simulink model "crop_simulation"  (R2021a)
settings: Solver=ode23tb  StartTime=0.0  StopTime=4  RelTol=1e-2
values from neighbouring files (symbols this model uses):
  parameters = LoadParameters()    [OnlyPlots.m]    (also in run_crop_simulation.m; run_several_crop_simulation.m)
undefined symbols (not defined in the file or in its folder): climate_GH3, MM_vec, nearst_p, p, PowerArtificial, Tr, Tref, Ts, x0_SOFC
libraries: HORTISIM x14, pid_lib x4
(part 2 of 3)

== system crop_simulation/Control Systems/Heater/SOFC/Subsystem2/Subsystem2 ==
  EPD : Inport
  Target : Inport  Port=2
  MATLAB Function : MATLAB Function  TreatAsAtomicUnit=on
  Memory : Memory
  Memory1 : Memory
  Rate Limiter : RateLimiter  RisingSlewLimit=5000  FallingSlewLimit=-5000
  Rate Transition : RateTransition  OutPortSampleTime=1/(60*24)
  Rate Transition1 : RateTransition  OutPortSampleTime=0
  Scope : Scope  NumInputPorts=3
  Vector Concatenate : Concatenate
  I [A] : Outport
  wires:
  MATLAB Function/1(y) -> Scope/2, Rate Transition1/1, Memory1/1
  EPD/1 -> Vector Concatenate/2, Memory/1
  Memory/1 -> Rate Transition/1
  Target/1 -> Vector Concatenate/1, MATLAB Function/1(Target)
  Rate Transition/1 -> MATLAB Function/2(FPD)
  Memory1/1 -> MATLAB Function/3(upre)
  Vector Concatenate/1 -> Scope/1
  Rate Limiter/1 -> Scope/3, I [A]/1
  Rate Transition1/1 -> Rate Limiter/1

== system crop_simulation/Control Systems/Heater/SOFC/Water Tank /Control Law ==
  Ti : Inport
  Tw : Inport  Port=2
  Constant : Constant  Value=273.15
  Control Flow Rate [%] : Subsystem
  Gain1 : Gain  Gain=90
  Minus : Sum  Inputs=+-
  Product : Product
  Scope2 : Scope
  Sum : Sum  Inputs=|++
  Heat[W] : Outport
  wires:
  Product/1 -> Heat[W]/1
  Tw/1 -> Minus/2
  Control Flow Rate [%]/1(Out1) -> Scope2/1, Product/2
  Gain1/1 -> Product/1
  Minus/1 -> Gain1/1
  Ti/1 -> Control Flow Rate [%]/1(Ti), Sum/1
  Sum/1 -> Minus/1
  Constant/1 -> Sum/2

== system crop_simulation/Control Systems/Heater/SOFC/Water Tank /recooling ==
  Tw : Inport
  Constant : Constant  Value=273.15 + 80
  Gain2 : Gain  Gain=500
  Minus1 : Sum  Inputs=+-
  Saturation : Saturate  UpperLimit=0  LowerLimit=-Inf  ZeroCross=off
  Qrecold : Outport
  wires:
  Constant/1 -> Minus1/1
  Tw/1 -> Minus1/2
  Saturation/1 -> Qrecold/1
  Minus1/1 -> Gain2/1
  Gain2/1 -> Saturation/1

== system crop_simulation/Control Systems/Heater/SOFC cascada/Battery/Calculo de Corriente atraves de la celda de combustible ==
  Target : Inport
  EPD : Inport  Port=2
  Continous : Subsystem  VariantControl=Choice_1
  Subsystem2 : Subsystem  VariantControl=Choice
      settings: PortSchema="{\"entries\":[{\"content\":{\"sides\":[{\"content\":{\"connectorIds\":[]},\"type\":\"ConnectorPlacement.EquallySpacedRectSide\",\"uuid\":\"50e66820-cd92-43dd-993d-153df9ce0354\"},{\"content\":{\"connectorIds\":[],\"side\":\"RIGHT\"},\"type\":\"ConnectorPlacement.EquallySpacedRectSide\",\"uuid\":\"8d846ca4-6643-48b0-8da4-4b4514e8854e\"},{\"content\":{\"connectorIds\":[\"Out1\"],\"side\":\"TOP\"},\"type\":\"ConnectorPlacement.EquallySpacedRectSide\",\"uuid\":\"89928db1-0ab3-4d04-989b-518ec70b2ccf\"},{\"content\":{\"connectorIds\":[\"In1\",\"In2\"],\"side\":\"BOTTOM\"},\"type\":\"ConnectorPlacement.EquallySpacedRectSide\",\"uuid\":\"be94ecfa-8f34-4f3e-bda2-4dff795f79cd\"}]},\"type\":\"ConnectorPlacement.EquallySpacedConnector\",\"uuid\":\"417f6773-c64e-42aa-b1d6-ce4fc249f7a2\"}],\"packageUris\":[\"http://schema.mathworks.com/mf0/Connector/R2020b\"],\"version\":\"1.0\"}"
  I [A] : Outport

== system crop_simulation/Control Systems/Heater/SOFC cascada/Control Operations Points/Control OP ==
  Tw_target [K] : Inport
  Tw [K] : Inport  Port=2
  Minus1 : Sum  Inputs=+-
  Scope : Scope  NumInputPorts=2
  Select Operation Point : Subsystem  Variant=on  VariantControlMode=label  VariantControl=Choice  LabelModeActiveChoice=Choice_2
  Transformacion Flujos : Subsystem
  Vector Concatenate : Concatenate
  OP : Outport
  wires:
  Transformacion Flujos/1(OP) -> OP/1
  Minus1/1 -> Select Operation Point/1(Error [ºC])
  Select Operation Point/1(OP) -> Scope/1, Transformacion Flujos/1(In1)  "OP"
  Tw_target [K]/1 -> Vector Concatenate/1, Minus1/1
  Vector Concatenate/1 -> Scope/2
  Tw [K]/1 -> Vector Concatenate/2, Minus1/2

== system crop_simulation/Control Systems/Heater/SOFC cascada/Control Operations Points/Control Tw ==
  Ti [ºC] : Inport
  Constant : Constant  Value=parameters.Tref
  Minus : Sum  Inputs=-+
  PID Controller : pid_lib/PID Controller  Controller=PID  Form=Parallel  TimeDomain=Continuous-time  UseExternalTs=off  SampleTime=-1  IntegratorMethod=Forward Euler  FilterMethod=Forward Euler  ControllerParametersSource=internal  P=50  I=1000  D=0  UseFilter=on  N=100  TunerSelectOption=Transfer Function Based (PID Tuner App)  InitialConditionSource=internal  InitialConditionForIntegrator=0  InitialConditionForFilter=0  DifferentiatorICPrevScaledInput=0  ExternalReset=none  TrackingMode=off  Kt=1  LimitOutput=on  SatLimitsSource=internal  UpperSaturationLimit=273.15 + 80  LowerSaturationLimit=273.15 + 60  LinearizeAsGain=on  AntiWindupMode=clamping  Kb=1  POutMin=[]  POutMax=[]  IOutMin=[]  IOutMax=[]  DOutMin=[]  DOutMax=[]  NOutMin=[]  NOutMax=[]  SumOutMin=[]  SumOutMax=[]  SaturationOutMin=[]  SaturationOutMax=[]  PParamMin=[]  PParamMax=[]  IParamMin=[]  IParamMax=[]  DParamMin=[]  DParamMax=[]  NParamMin=[]  NParamMax=[]  KbParamMin=[]  KbParamMax=[]  KtParamMin=[]  KtParamMax=[]  KbOutMin=[]  KbOutMax=[]  KtOutMin=[]  KtOutMax=[]  IntegratorOutMin=[]  IntegratorOutMax=[]  FilterOutMin=[]  FilterOutMax=[]  SumI1OutMin=[]  SumI1OutMax=[]  SumI2OutMin=[]  SumI2OutMax=[]  SumI3OutMin=[]  SumI3OutMax=[]  SumI4OutMin=[]  SumI4OutMax=[]  SumDOutMin=[]  SumDOutMax=[]  DifferentiatorOutMin=[]  DifferentiatorOutMax=[]  FilterDiffOutCoefMin=[]  FilterDiffOutCoefMax=[]  ReciprocalOutMin=[]  ReciprocalOutMax=[]  SumDenOutMin=[]  SumDenOutMax=[]  SumNumOutMin=[]  SumNumOutMax=[]  DivideOutMin=[]  DivideOutMax=[]  UdiffTsProdOutMin=[]  UdiffTsProdOutMax=[]  NTsProdOutMin=[]  NTsProdOutMax=[]  UintegralTsProdOutMin=[]  UintegralTsProdOutMax=[]  UngainTsProdOutMin=[]  UngainTsProdOutMax=[]  IntegratorContinuousStateAttributes=''  IntegratorStateMustResolveToSignalObject=off  IntegratorRTWStateStorageClass=Auto  FilterContinuousStateAttributes=''  FilterStateMustResolveToSignalObject=off  FilterRTWStateStorageClass=Auto  ParallelPVariant=InternalParameters  IdealPVariant=Disabled  IVariant=InternalParameters  DVariant=InternalParameters  IntegratorVariant=Continuous  SatVariant=Enabled  AWVariant=ContClampingParallel  PCopyVariant=Disabled  TRVariant=Disabled  FdbkBlocksVariant=Forward  IdealPFdbkVariant=Disabled  SatFdbkVariant=Disabled  DerivativeFilterVariant=ContFilter  NVariant=InternalParameters  NCopyVariant=Disabled  FilterICVariant=InternalICsFilter  IntegratorICVariant=InternalICs  ExternalResetVariant=Disabled  TRSumVariant=Passthrough  SumFdbkVariant=Disabled  SumVariant=Sum_PID  TsampFilterVariant=InternalTs  TsampNgainVariant=Passthrough  TsampIntegralVariant=Passthrough  ExternalSaturationOutDataTypeStr=Inherit: Same as second input
  Scope : Scope  NumInputPorts=2
  Vector Concatenate : Concatenate
  Tw_target [K] : Outport
  wires:
  Constant/1 -> Minus/2, Vector Concatenate/2
  Minus/1 -> PID Controller/1
  PID Controller/1 -> Scope/2, Tw_target [K]/1
  Ti [ºC]/1 -> Vector Concatenate/1, Minus/1
  Vector Concatenate/1 -> Scope/1

== system crop_simulation/Control Systems/Heater/SOFC cascada/Electrical Heating Rod/If Action Subsystem ==
  Action Port : ActionPort  ActionPortLabel=if(u1 < 1)
  Constant : Constant  Value=200
  Out1 : Outport
  wires:
  Constant/1 -> Out1/1

== system crop_simulation/Control Systems/Heater/SOFC cascada/Electrical Heating Rod/If Action Subsystem1 ==
  Action Port : ActionPort  ActionPortLabel=else
  Constant : Constant  Value=0
  Out1 : Outport
  wires:
  Constant/1 -> Out1/1

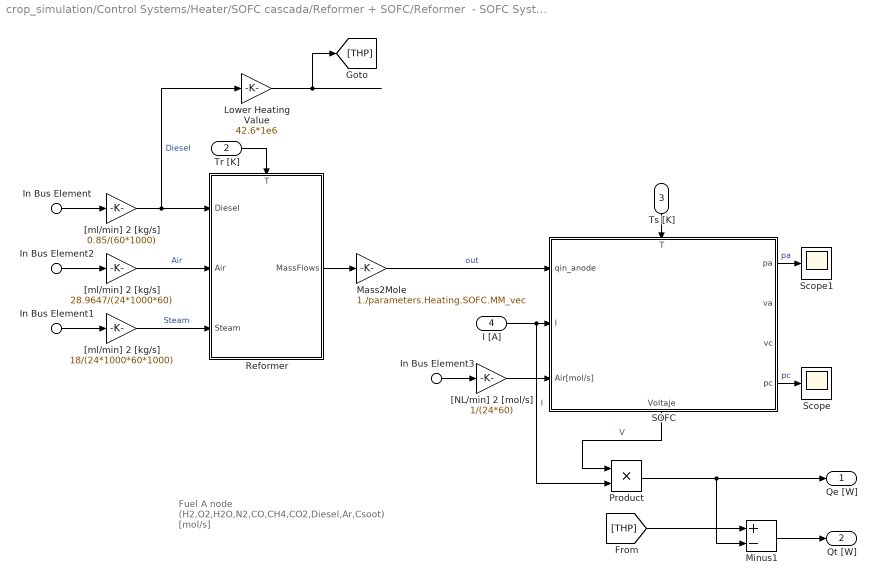
== system crop_simulation/Control Systems/Heater/SOFC cascada/Reformer + SOFC/Reformer  - SOFC System ==
  note: Fuel
      | A node
      | (H2,O2,H2O,N2,CO,CH4,CO2,Diesel,Ar,Csoot)
      | [mol/s]
  In Bus Element : Inport  PortName=OP  Element=Diesel [ml/min]
  In Bus Element1 : Inport  PortName=OP  Element=Steam [ml/min]
  In Bus Element2 : Inport  PortName=OP  Element=Air [NL/min]
  In Bus Element3 : Inport  PortName=OP  Element=Air_cath [NL/min]
  Tr [K] : Inport  Port=2
  Ts [K] : Inport  Port=3
  I [A] : Inport  Port=4
  Lower Heating Value : Gain  Gain=42.6*1e6
  Mass2Mole : Gain  Gain=1./parameters.Heating.SOFC.MM_vec
  Minus1 : Sum  Inputs=+-
  Product : Product
  "Reformer " : Subsystem
      settings: PortSchema="{\"entries\":[{\"content\":{\"sides\":[{\"content\":{\"connectorIds\":[\"In1\",\"In2\",\"In3\"]},\"type\":\"ConnectorPlacement.EquallySpacedRectSide\",\"uuid\":\"bf799419-3c51-4e41-80c3-8f053955be8d\"},{\"content\":{\"connectorIds\":[\"Out1\"],\"side\":\"RIGHT\"},\"type\":\"ConnectorPlacement.EquallySpacedRectSide\",\"uuid\":\"8203b5dc-5749-4c6f-8169-46d2df527b78\"},{\"content\":{\"connectorIds\":[\"In4\"],\"side\":\"TOP\"},\"type\":\"ConnectorPlacement.EquallySpacedRectSide\",\"uuid\":\"29bf5c31-2b54-418d-a6d2-10fc76893a8c\"}]},\"type\":\"ConnectorPlacement.EquallySpacedConnector\",\"uuid\":\"ce77c350-1f9b-4f0b-aae0-5de0ba71c7e8\"}],\"packageUris\":[\"http://schema.mathworks.com/mf0/Connector/R2020b\"],\"version\":\"1.0\"}"
  "SOFC " : Subsystem  mask{p=parameters.Heating.SOFC.params, x0=parameters.Heating.SOFC.x0, nearst_p=parameters.Heating.SOFC.nearst_p}
      mask prompts: p "params"
      settings: PortSchema="{\"entries\":[{\"content\":{\"sides\":[{\"content\":{\"connectorIds\":[\"In1\",\"In2\",\"In3\"]},\"type\":\"ConnectorPlacement.EquallySpacedRectSide\",\"uuid\":\"6cca8e4f-6db2-48de-a60a-b6fbc16877c6\"},{\"content\":{\"connectorIds\":[\"Out1\",\"Out2\",\"Out3\",\"Out4\"],\"side\":\"RIGHT\"},\"type\":\"ConnectorPlacement.EquallySpacedRectSide\",\"uuid\":\"c481f6d1-531d-4215-9ae0-5807376c0625\"},{\"content\":{\"connectorIds\":[\"In4\"],\"side\":\"TOP\"},\"type\":\"ConnectorPlacement.EquallySpacedRectSide\",\"uuid\":\"76720726-927e-4340-b17d-e33f4db2c782\"},{\"content\":{\"connectorIds\":[\"Out5\"],\"side\":\"BOTTOM\"},\"type\":\"ConnectorPlacement.EquallySpacedRectSide\",\"uuid\":\"7ed108e3-6588-44d6-8f3d-9789ffe258a7\"}]},\"type\":\"ConnectorPlacement.EquallySpacedConnector\",\"uuid\":\"f9228f26-0840-43d6-932a-2fdb8a27bf20\"}],\"packageUris\":[\"http://schema.mathworks.com/mf0/Connector/R2020b\"],\"version\":\"1.0\"}"
  Scope : Scope
  Scope1 : Scope
  "[NL/min] 2 [mol/s]" : Gain  Gain=1/(24*60)
  "[ml/min] 2 [kg/s]" : Gain  Gain=0.85/(60*1000)
  "[ml/min] 2 [kg/s] " : Gain  Gain=28.9647/(24*1000*60)
  "[ml/min] 2 [kg/s]  " : Gain  Gain=18/(24*1000*60*1000)
  Qe [W] : Outport
  Qt [W] : Outport  Port=2
  wires:
  I [A]/1 -> "SOFC "/2(I), Product/2  "I"
  "SOFC "/5(Voltaje) -> Product/1  "V"
  Ts [K]/1 -> "SOFC "/4(T)
  Product/1 -> Qe [W]/1, Minus1/2
  In Bus Element/1 -> "[ml/min] 2 [kg/s]"/1
  In Bus Element2/1 -> "[ml/min] 2 [kg/s] "/1
  In Bus Element1/1 -> "[ml/min] 2 [kg/s]  "/1
  In Bus Element3/1 -> "[NL/min] 2 [mol/s]"/1
  "[NL/min] 2 [mol/s]"/1 -> "SOFC "/3(Air[mol/s])
  Lower Heating Value/1 -> [THP]
  [THP] -> Minus1/1
  Minus1/1 -> Qt [W]/1
  "SOFC "/4(pc) -> Scope/1  "pc"
  "SOFC "/1(pa) -> Scope1/1  "pa"
  "Reformer "/1(MassFlows) -> Mass2Mole/1
  Tr [K]/1 -> "Reformer "/4(T)
  "[ml/min] 2 [kg/s]"/1 -> Lower Heating Value/1, "Reformer "/1(Diesel)  "Diesel"
  "[ml/min] 2 [kg/s] "/1 -> "Reformer "/2(Air)  "Air"
  "[ml/min] 2 [kg/s]  "/1 -> "Reformer "/3(Steam)  "Steam"
  Mass2Mole/1 -> "SOFC "/1(qin_anode)  "out"

== system crop_simulation/Control Systems/Heater/SOFC cascada/Water Tank /Control Law ==
  Ti : Inport
  Tw : Inport  Port=2
  Constant : Constant  Value=273.15
  Control Flow Rate [%] : Subsystem
  Gain1 : Gain  Gain=90
  Minus : Sum  Inputs=+-
  Product : Product
  Scope2 : Scope
  Sum : Sum  Inputs=|++
  Heat[W] : Outport
  wires:
  Product/1 -> Heat[W]/1
  Tw/1 -> Minus/2
  Control Flow Rate [%]/1(Out1) -> Scope2/1, Product/2
  Gain1/1 -> Product/1
  Minus/1 -> Gain1/1
  Ti/1 -> Control Flow Rate [%]/1(Ti), Sum/1
  Sum/1 -> Minus/1
  Constant/1 -> Sum/2

== system crop_simulation/Control Systems/Heater/SOFC cascada/Water Tank /recooling ==
  Tw : Inport
  Constant : Constant  Value=273.15 + 80
  Gain2 : Gain  Gain=500
  Minus1 : Sum  Inputs=+-
  Saturation : Saturate  UpperLimit=0  LowerLimit=-Inf  ZeroCross=off
  Qrecold : Outport
  wires:
  Constant/1 -> Minus1/1
  Tw/1 -> Minus1/2
  Saturation/1 -> Qrecold/1
  Minus1/1 -> Gain2/1
  Gain2/1 -> Saturation/1

== system crop_simulation/Control Systems/Heater/SOFC/Control OP/Select Operation Point/Relay ==
  Tw [ºC] : Inport
  Relay : Relay  OnSwitchValue=80  OffSwitchValue=20  OnOutputValue=2  OffOutputValue=4
  OP : Outport
  wires:
  Tw [ºC]/1 -> Relay/1
  Relay/1 -> OP/1

== system crop_simulation/Control Systems/Heater/SOFC/Control OP/Select Operation Point/Relay 3 ==
  Tw [ºC] : Inport
  Delay : Delay  DelayLength=1  InitialCondition=1
  MATLAB Function : MATLAB Function  TreatAsAtomicUnit=on
  Rate Transition : RateTransition  InitialCondition=10  OutPortSampleTime=1/(60*24)
  OP : Outport
  wires:
  MATLAB Function/1(next_state) -> Delay/1, OP/1
  Delay/1 -> MATLAB Function/2(state)
  Tw [ºC]/1 -> Rate Transition/1
  Rate Transition/1 -> MATLAB Function/1(Tw)

== system crop_simulation/Control Systems/Heater/SOFC/Control OP/Select Operation Point/Select Operation Point ==
  Tw [ºC] : Inport
  If : If  IfExpression=u1 < 20  ElseIfExpressions=(u1 >= 20)&(u1<50),u1>=50  ShowElse=off  ZeroCross=off
  If Action Subsystem : Subsystem  TreatAsAtomicUnit=on
  If Action Subsystem1 : Subsystem  TreatAsAtomicUnit=on
  If Action Subsystem2 : Subsystem  TreatAsAtomicUnit=on
  Merge : Merge  Inputs=3
  OP : Outport
  wires:
  Tw [ºC]/1 -> If/1
  If Action Subsystem1/1(Out1) -> Merge/2
  Merge/1 -> OP/1
  If/3 -> If Action Subsystem2/Action
  If/1 -> If Action Subsystem/Action
  If Action Subsystem2/1(Out1) -> Merge/3
  If Action Subsystem/1(Out1) -> Merge/1
  If/2 -> If Action Subsystem1/Action

== system crop_simulation/Control Systems/Heater/SOFC/Control OP/Transformacion Flujos/If Action Subsystem ==
  Action Port : ActionPort  ActionPortLabel=case [ 4 ]:
  Subsystem : Subsystem
  Out1 : Outport
  wires:
  Subsystem/1(OP) -> Out1/1

== system crop_simulation/Control Systems/Heater/SOFC/Control OP/Transformacion Flujos/If Action Subsystem1 ==
  Action Port : ActionPort  ActionPortLabel=case [ 3 ]:
  Subsystem1 : Subsystem
  Out1 : Outport
  wires:
  Subsystem1/1(OP) -> Out1/1

== system crop_simulation/Control Systems/Heater/SOFC/Control OP/Transformacion Flujos/If Action Subsystem2 ==
  Action Port : ActionPort  ActionPortLabel=case [ 2 ]:
  Subsystem2 : Subsystem
  Out1 : Outport
  wires:
  Subsystem2/1(OP) -> Out1/1

== system crop_simulation/Control Systems/Heater/SOFC/Control OP/Transformacion Flujos/If Action Subsystem3 ==
  Action Port : ActionPort  ActionPortLabel=case [ 1 ]:
  Subsystem2 : Subsystem
  Out1 : Outport
  wires:
  Subsystem2/1(OP) -> Out1/1

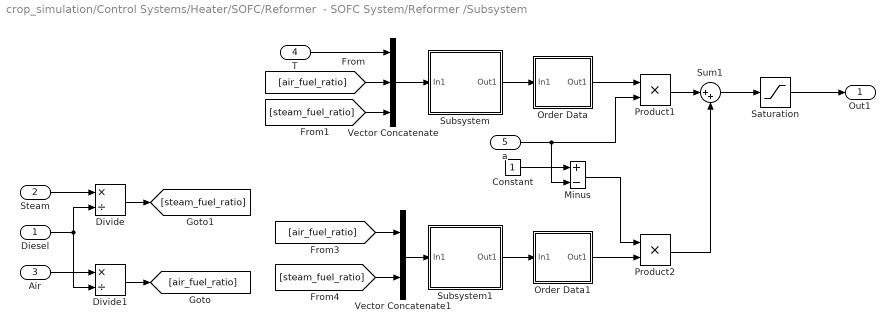
== system crop_simulation/Control Systems/Heater/SOFC/Reformer  - SOFC System/Reformer /Subsystem ==
  Diesel : Inport
  Steam : Inport  Port=2
  Air : Inport  Port=3
  T : Inport  Port=4
  a : Inport  Port=5
  Constant : Constant
  Divide : Product  Inputs=*/
  Divide1 : Product  Inputs=*/
  Minus : Sum  Inputs=+-
  Order Data : Subsystem
  Order Data1 : Subsystem
  Product1 : Product
  Product2 : Product
  Saturation : Saturate  UpperLimit=inf  LowerLimit=0
  Subsystem : Subsystem  Variant=on  VariantControlMode=label  VariantControl=Choice  LabelModeActiveChoice=Choice_1
  Subsystem1 : Subsystem  Variant=on  VariantControlMode=label  VariantControl=Choice  LabelModeActiveChoice=Choice_1
  Sum1 : Sum  Inputs=|++
  Vector Concatenate : Concatenate  NumInputs=3
  Vector Concatenate1 : Concatenate
  Out1 : Outport
  wires:
  a/1 -> Product1/2, Minus/2
  [steam_fuel_ratio] -> Vector Concatenate/3
  Product1/1 -> Sum1/1
  T/1 -> Vector Concatenate/1
  [air_fuel_ratio] -> Vector Concatenate1/1
  Product2/1 -> Sum1/2
  [steam_fuel_ratio] -> Vector Concatenate1/2
  Order Data1/1(Out1) -> Product2/2
  Minus/1 -> Product2/1
  Order Data/1(Out1) -> Product1/1
  [air_fuel_ratio] -> Vector Concatenate/2
  Constant/1 -> Minus/1
  Steam/1 -> Divide/1
  Diesel/1 -> Divide1/2, Divide/2
  Air/1 -> Divide1/1
  Divide/1 -> [steam_fuel_ratio]
  Divide1/1 -> [air_fuel_ratio]
  Saturation/1 -> Out1/1
  Sum1/1 -> Saturation/1
  Vector Concatenate/1 -> Subsystem/1(In1)
  Subsystem/1(Out1) -> Order Data/1(In1)
  Vector Concatenate1/1 -> Subsystem1/1(In1)
  Subsystem1/1(Out1) -> Order Data1/1(In1)

== system crop_simulation/Control Systems/Heater/SOFC/Reformer  - SOFC System/SOFC /Anode ==
  qa_in : Inport
  I : Inport  Port=2
  pc_O2 : Inport  Port=3
  T : Inport  Port=4
  Divide2 : Product  Inputs=**
  Gain : Gain  Gain=p.ValveConstants_an
  Gain1 : Gain  Gain=p.N0
  Gain2 : Gain  Gain=p.R/p.Vanode
  Integrator : Integrator  InitialCondition=x0_SOFC.pa  LowerSaturationLimit=0  ZeroCross=off
  MATLAB Function : MATLAB Function  TreatAsAtomicUnit=on
  Scope : Scope
  Scope1 : Scope
  Scope2 : Scope
  Sum : Sum  Inputs=+-+
  seconds 2 days : Gain  Gain=3600*24
  pa : Outport
  pa_out : Outport  Port=2
  la : Outport  Port=3
  wires:
  Sum/1 -> Divide2/1
  Integrator/1 -> Scope/1, Gain/1, MATLAB Function/4(pa), pa/1
  Gain2/1 -> Divide2/2
  qa_in/1 -> Sum/1, MATLAB Function/1(qa_in)
  Gain/1 -> pa_out/1, Sum/2
  I/1 -> MATLAB Function/2(I)
  T/1 -> Gain2/1
  MATLAB Function/2(la) -> la/1, Scope1/1
  pc_O2/1 -> MATLAB Function/3(pc_O2)
  MATLAB Function/1(ra) -> Gain1/1
  Gain1/1 -> Scope2/1, Sum/3
  Divide2/1 -> seconds 2 days/1
  seconds 2 days/1 -> Integrator/1

== system crop_simulation/Control Systems/Heater/SOFC/Reformer  - SOFC System/SOFC /Cathode ==
  qc_in : Inport
  I : Inport  Port=2
  T : Inport  Port=3
  Divide3 : Product  Inputs=**
  Gain1 : Gain  Gain=p.N0
  Gain2 : Gain  Gain=p.R/p.Vcatho
  Integrator1 : Integrator  InitialCondition=x0_SOFC.pc  LowerSaturationLimit=0  ZeroCross=off
  MATLAB Function : MATLAB Function  TreatAsAtomicUnit=on
  Scope : Scope
  Scope1 : Scope  NumInputPorts=2
  Selector : Selector  InputPortWidth=10  IndexOptions=Index vector (dialog)  Indices=2  OutputSizes=1
  Sum1 : Sum  Inputs=+-+
  seconds 2 days : Gain  Gain=3600*24
  valve : Gain  Gain=p.ValveConstants_cath
  pc : Outport
  pc_out : Outport  Port=2  Unit=mol/s
  pc_O2 : Outport  Port=3
  wires:
  Sum1/1 -> Divide3/1
  Integrator1/1 -> Selector/1, valve/1, Scope/1, pc/1
  qc_in/1 -> Sum1/1
  Gain2/1 -> Divide3/2
  T/1 -> Gain2/1
  valve/1 -> Sum1/2, pc_out/1
  I/1 -> Scope1/1, MATLAB Function/1(I)
  MATLAB Function/1(rc) -> Gain1/1
  Gain1/1 -> Sum1/3
  Divide3/1 -> seconds 2 days/1
  seconds 2 days/1 -> Integrator1/1
  Selector/1 -> pc_O2/1, Scope1/2, MATLAB Function/2(pc_O2)

== system crop_simulation/Control Systems/Heater/SOFC/Reformer  - SOFC System/SOFC /Nernst’s Eq  ==
  note: Hemos fijado la dimension de salida de este bloque
  note: 'H2' , 'O2' , 'H2O' , 'N2' , 'CO' , 'CH4' , 'CO2' , 'Diesel' ,'Ar','Csoot'
  Xa : Inport
  I : Inport  Port=2
  T : Inport  Port=3
  ratio a/c : Inport  Port=4
  Constant5 : Constant  Value=nearst_p.mu_out
  Gain : Gain  Gain=nearst_p.std_out
  MATLAB Function1 : MATLAB Function  TreatAsAtomicUnit=on
  Scope1 : Scope
  Subsystem : Subsystem
  Subsystem1 : Subsystem  Variant=on  VariantControlMode=label  VariantControl=Choice  LabelModeActiveChoice=Choice_1
  Sum : Sum  Inputs=|++
  V : Outport  PortDimensions=1
  wires:
  T/1 -> Subsystem/2(T)
  Xa/1 -> Subsystem/3(la)
  ratio a/c/1 -> Subsystem/1(ratio a/c)
  Gain/1 -> Sum/1
  Constant5/1 -> Sum/2
  Sum/1 -> Scope1/1, MATLAB Function1/1(params)
  MATLAB Function1/1(V) -> V/1
  I/1 -> MATLAB Function1/2(I)
  Subsystem/1(Out7) -> Subsystem1/1(In1)
  Subsystem1/1(Out1) -> Gain/1

== system crop_simulation/Control Systems/Heater/SOFC/Reformer  - SOFC System/SOFC /Subsystem ==
  Air[mol/s] : Inport
  Molar Fractions (H2,O2,H2O,N2,CO,CH4,CO2) [mol/(Air-mol)] : Constant  Value=[0 0.2095 0 0.7808 0 0 0 0 0 0]
  Product : Product
  Cathode [mol/s] : Outport
  wires:
  Air[mol/s]/1 -> Product/1  "Air [mol/s]"
  Product/1 -> Cathode [mol/s]/1  "Cathode [mol/s]"
  Molar Fractions (H2,O2,H2O,N2,CO,CH4,CO2) [mol/(Air-mol)]/1 -> Product/2

== system crop_simulation/Control Systems/Heater/SOFC/Water Tank /Control Law/Control Flow Rate [%] ==
  Ti : Inport
  Constant : Constant  Value=Tref
  Minus : Sum  Inputs=+-
  PID Controller : pid_lib/PID Controller  Controller=PID  Form=Parallel  TimeDomain=Continuous-time  UseExternalTs=off  SampleTime=-1  IntegratorMethod=Forward Euler  FilterMethod=Forward Euler  ControllerParametersSource=internal  P=1.5  I=1  D=0  UseFilter=on  N=100  TunerSelectOption=Transfer Function Based (PID Tuner App)  InitialConditionSource=internal  InitialConditionForIntegrator=0  InitialConditionForFilter=0  DifferentiatorICPrevScaledInput=0  ExternalReset=none  TrackingMode=off  Kt=1  LimitOutput=on  SatLimitsSource=internal  UpperSaturationLimit=1  LowerSaturationLimit=0  LinearizeAsGain=on  AntiWindupMode=clamping  Kb=1  POutMin=[]  POutMax=[]  IOutMin=[]  IOutMax=[]  DOutMin=[]  DOutMax=[]  NOutMin=[]  NOutMax=[]  SumOutMin=[]  SumOutMax=[]  SaturationOutMin=[]  SaturationOutMax=[]  PParamMin=[]  PParamMax=[]  IParamMin=[]  IParamMax=[]  DParamMin=[]  DParamMax=[]  NParamMin=[]  NParamMax=[]  KbParamMin=[]  KbParamMax=[]  KtParamMin=[]  KtParamMax=[]  KbOutMin=[]  KbOutMax=[]  KtOutMin=[]  KtOutMax=[]  IntegratorOutMin=[]  IntegratorOutMax=[]  FilterOutMin=[]  FilterOutMax=[]  SumI1OutMin=[]  SumI1OutMax=[]  SumI2OutMin=[]  SumI2OutMax=[]  SumI3OutMin=[]  SumI3OutMax=[]  SumI4OutMin=[]  SumI4OutMax=[]  SumDOutMin=[]  SumDOutMax=[]  DifferentiatorOutMin=[]  DifferentiatorOutMax=[]  FilterDiffOutCoefMin=[]  FilterDiffOutCoefMax=[]  ReciprocalOutMin=[]  ReciprocalOutMax=[]  SumDenOutMin=[]  SumDenOutMax=[]  SumNumOutMin=[]  SumNumOutMax=[]  DivideOutMin=[]  DivideOutMax=[]  UdiffTsProdOutMin=[]  UdiffTsProdOutMax=[]  NTsProdOutMin=[]  NTsProdOutMax=[]  UintegralTsProdOutMin=[]  UintegralTsProdOutMax=[]  UngainTsProdOutMin=[]  UngainTsProdOutMax=[]  IntegratorContinuousStateAttributes=''  IntegratorStateMustResolveToSignalObject=off  IntegratorRTWStateStorageClass=Auto  FilterContinuousStateAttributes=''  FilterStateMustResolveToSignalObject=off  FilterRTWStateStorageClass=Auto  ParallelPVariant=InternalParameters  IdealPVariant=Disabled  IVariant=InternalParameters  DVariant=InternalParameters  IntegratorVariant=Continuous  SatVariant=Enabled  AWVariant=ContClampingParallel  PCopyVariant=Disabled  TRVariant=Disabled  FdbkBlocksVariant=Forward  IdealPFdbkVariant=Disabled  SatFdbkVariant=Disabled  DerivativeFilterVariant=ContFilter  NVariant=InternalParameters  NCopyVariant=Disabled  FilterICVariant=InternalICsFilter  IntegratorICVariant=InternalICs  ExternalResetVariant=Disabled  TRSumVariant=Passthrough  SumFdbkVariant=Disabled  SumVariant=Sum_PID  TsampFilterVariant=InternalTs  TsampNgainVariant=Passthrough  TsampIntegralVariant=Passthrough  ExternalSaturationOutDataTypeStr=Inherit: Same as second input
  Scope : Scope  NumInputPorts=2
  Out1 : Outport
  wires:
  Constant/1 -> Scope/1, Minus/1
  Minus/1 -> PID Controller/1
  Ti/1 -> Scope/2, Minus/2
  PID Controller/1 -> Out1/1

== system crop_simulation/Control Systems/Heater/SOFC cascada/Battery/Calculo de Corriente atraves de la celda de combustible/Continous ==
  Target : Inport
  EPD : Inport  Port=2
  Gain : Gain  Gain=24*3600*0.01
  Integrator : Integrator  InitialCondition=10  LimitOutput=on  UpperSaturationLimit=30  LowerSaturationLimit=1
  Minus : Sum  Inputs=+-
  Scope : Scope  NumInputPorts=2
  Vector Concatenate : Concatenate
  I [A] : Outport
  wires:
  Target/1 -> Minus/1, Vector Concatenate/1
  EPD/1 -> Vector Concatenate/2, Minus/2
  Integrator/1 -> Scope/1, I [A]/1
  Gain/1 -> Integrator/1
  Minus/1 -> Gain/1
  Vector Concatenate/1 -> Scope/2

== system crop_simulation/Control Systems/Heater/SOFC cascada/Battery/Calculo de Corriente atraves de la celda de combustible/Subsystem2 ==
  EPD : Inport
  Target : Inport  Port=2
  MATLAB Function : MATLAB Function  TreatAsAtomicUnit=on
  Memory : Memory
  Memory1 : Memory
  Rate Limiter : RateLimiter  RisingSlewLimit=5000  FallingSlewLimit=-5000
  Rate Transition : RateTransition  OutPortSampleTime=1/(60*24)
  Rate Transition1 : RateTransition  OutPortSampleTime=0
  Scope : Scope  NumInputPorts=3
  Vector Concatenate : Concatenate
  I [A] : Outport
  wires:
  MATLAB Function/1(y) -> Scope/2, Rate Transition1/1, Memory1/1
  EPD/1 -> Vector Concatenate/2, Memory/1
  Memory/1 -> Rate Transition/1
  Target/1 -> Vector Concatenate/1, MATLAB Function/1(Target)
  Rate Transition/1 -> MATLAB Function/2(FPD)
  Memory1/1 -> MATLAB Function/3(upre)
  Vector Concatenate/1 -> Scope/1
  Rate Limiter/1 -> Scope/3, I [A]/1
  Rate Transition1/1 -> Rate Limiter/1

== system crop_simulation/Control Systems/Heater/SOFC cascada/Control Operations Points/Control OP/Select Operation Point ==
  Error [ºC] : Inport
  Relay : Subsystem  VariantControl=Choice_1
  Relay 3 : Subsystem  VariantControl=Choice_2
  Select Operation Point : Subsystem  VariantControl=Choice
  OP : Outport

== system crop_simulation/Control Systems/Heater/SOFC cascada/Control Operations Points/Control OP/Transformacion Flujos ==
  In1 : Inport
  If Action Subsystem : Subsystem  TreatAsAtomicUnit=on
  If Action Subsystem1 : Subsystem  TreatAsAtomicUnit=on
  If Action Subsystem2 : Subsystem  TreatAsAtomicUnit=on
  If Action Subsystem3 : Subsystem  TreatAsAtomicUnit=on
  Merge : Merge  Inputs=4
  Rate Limiter : RateLimiter  RisingSlewLimit=500  FallingSlewLimit=-500  SampleTimeMode=inherited
  Scope : Scope  NumInputPorts=2
  Switch Case : SwitchCase  CaseConditions={4,3,2,1}  ShowDefaultCase=off
  OP : Outport
  wires:
  In1/1 -> Switch Case/1
  Switch Case/3 -> If Action Subsystem2/Action
  If Action Subsystem1/1(Out1) -> Merge/2
  If Action Subsystem/1(Out1) -> Merge/1
  If Action Subsystem2/1(Out1) -> Merge/3
  Merge/1 -> Scope/2, Rate Limiter/1, OP/1
  Switch Case/2 -> If Action Subsystem1/Action
  Switch Case/1 -> If Action Subsystem/Action
  Switch Case/4 -> If Action Subsystem3/Action
  If Action Subsystem3/1(Out1) -> Merge/4
  Rate Limiter/1 -> Scope/1

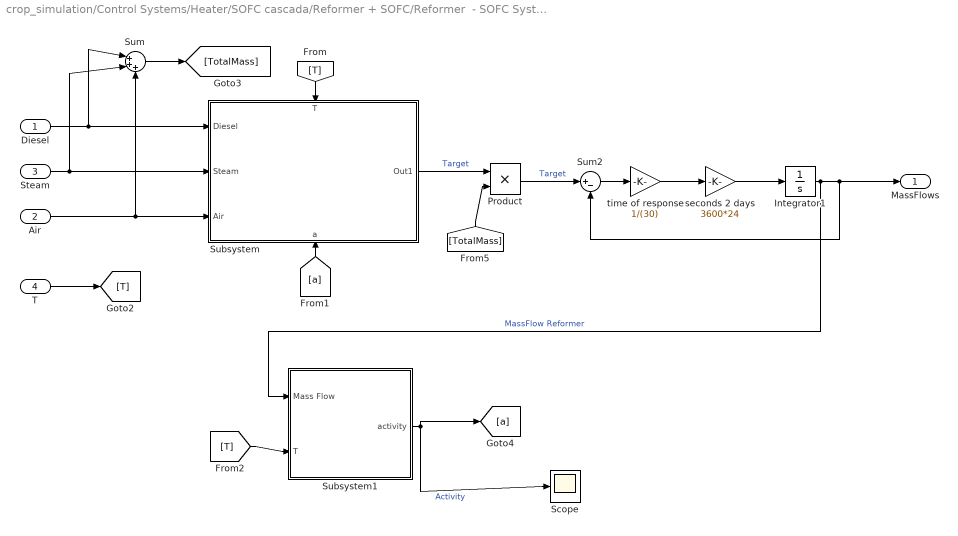
== system crop_simulation/Control Systems/Heater/SOFC cascada/Reformer + SOFC/Reformer  - SOFC System/Reformer  ==
  Diesel : Inport
  Air : Inport  Port=2
  Steam : Inport  Port=3
  T : Inport  Port=4
  Integrator1 : Integrator  InitialCondition=1e-6
  Product : Product
  Scope : Scope
  Subsystem : Subsystem
      settings: PortSchema="{\"entries\":[{\"content\":{\"sides\":[{\"content\":{\"connectorIds\":[\"In1\",\"In2\",\"In3\"]},\"type\":\"ConnectorPlacement.EquallySpacedRectSide\",\"uuid\":\"0dada652-6957-4c3e-8e48-73ee360a3bab\"},{\"content\":{\"connectorIds\":[\"Out1\"],\"side\":\"RIGHT\"},\"type\":\"ConnectorPlacement.EquallySpacedRectSide\",\"uuid\":\"81208621-951c-43f9-b655-3502a16ce57a\"},{\"content\":{\"connectorIds\":[\"In4\"],\"side\":\"TOP\"},\"type\":\"ConnectorPlacement.EquallySpacedRectSide\",\"uuid\":\"1012e2be-7d0b-44a9-9a40-bc453950010e\"},{\"content\":{\"connectorIds\":[\"In5\"],\"side\":\"BOTTOM\"},\"type\":\"ConnectorPlacement.EquallySpacedRectSide\",\"uuid\":\"aaef83a2-abb7-4780-82b5-9abad57d39ad\"}]},\"type\":\"ConnectorPlacement.EquallySpacedConnector\",\"uuid\":\"1143871f-aacc-4fa7-a444-9910d5016eff\"}],\"packageUris\":[\"http://schema.mathworks.com/mf0/Connector/R2020b\"],\"version\":\"1.0\"}"
  Subsystem1 : Subsystem  Variant=on  VariantControlMode=label  VariantControl=Choice  LabelModeActiveChoice=Choice_1
  Sum : Sum  Inputs=|+++
  Sum2 : Sum  Inputs=|+-
  seconds 2 days : Gain  Gain=3600*24
  time of response : Gain  Gain=1/(30)
  MassFlows : Outport
  wires:
  T/1 -> [T]
  Sum/1 -> [TotalMass]
  [TotalMass] -> Product/2
  Diesel/1 -> Subsystem/1(Diesel), Sum/1
  [a] -> Subsystem/5(a)
  [T] -> Subsystem/4(T)
  time of response/1 -> seconds 2 days/1
  Sum2/1 -> time of response/1
  Product/1 -> Sum2/1  "Target"
  seconds 2 days/1 -> Integrator1/1
  Integrator1/1 -> MassFlows/1, Sum2/2, Subsystem1/1(Mass Flow)  "MassFlow Reformer"
  Subsystem/1(Out1) -> Product/1  "Target"
  Steam/1 -> Subsystem/2(Steam), Sum/2
  Air/1 -> Subsystem/3(Air), Sum/3
  Subsystem1/1(activity) -> Scope/1, [a]  "Activity"
  [T] -> Subsystem1/2(T)

== system crop_simulation/Control Systems/Heater/SOFC cascada/Reformer + SOFC/Reformer  - SOFC System/SOFC  ==
  qin_anode : Inport
  I : Inport  Port=2
  Air[mol/s] : Inport  Port=3
  T : Inport  Port=4
  Anode : Subsystem
      settings: PortSchema="{\"entries\":[{\"content\":{\"sides\":[{\"content\":{\"connectorIds\":[\"In1\"]},\"type\":\"ConnectorPlacement.EquallySpacedRectSide\",\"uuid\":\"1d27f661-9cb9-482d-ac43-89e84d52643b\"},{\"content\":{\"connectorIds\":[\"Out1\",\"Out2\",\"Out3\"],\"side\":\"RIGHT\"},\"type\":\"ConnectorPlacement.EquallySpacedRectSide\",\"uuid\":\"62ac897d-5819-4e9c-a19f-e210851aefa2\"},{\"content\":{\"connectorIds\":[],\"side\":\"TOP\"},\"type\":\"ConnectorPlacement.EquallySpacedRectSide\",\"uuid\":\"1380e9d4-c5ac-42ce-b6fc-00336cc8edba\"},{\"content\":{\"connectorIds\":[\"In2\",\"In3\",\"In4\"],\"side\":\"BOTTOM\"},\"type\":\"ConnectorPlacement.EquallySpacedRectSide\",\"uuid\":\"0e36fd1a-38eb-48cb-8834-06d558b43614\"}]},\"type\":\"ConnectorPlacement.EquallySpacedConnector\",\"uuid\":\"79a72313-dbdc-4de5-b88f-787bafe984c7\"}],\"packageUris\":[\"http://schema.mathworks.com/mf0/Connector/R2020b\"],\"version\":\"1.0\"}"
  Cathode : Subsystem
      settings: PortSchema="{\"entries\":[{\"content\":{\"sides\":[{\"content\":{\"connectorIds\":[\"In1\"]},\"type\":\"ConnectorPlacement.EquallySpacedRectSide\",\"uuid\":\"1d27f661-9cb9-482d-ac43-89e84d52643b\"},{\"content\":{\"connectorIds\":[\"Out1\",\"Out2\"],\"side\":\"RIGHT\"},\"type\":\"ConnectorPlacement.EquallySpacedRectSide\",\"uuid\":\"62ac897d-5819-4e9c-a19f-e210851aefa2\"},{\"content\":{\"connectorIds\":[\"In2\",\"Out3\",\"In3\"],\"side\":\"TOP\"},\"type\":\"ConnectorPlacement.EquallySpacedRectSide\",\"uuid\":\"1380e9d4-c5ac-42ce-b6fc-00336cc8edba\"}]},\"type\":\"ConnectorPlacement.EquallySpacedConnector\",\"uuid\":\"79a72313-dbdc-4de5-b88f-787bafe984c7\"}],\"packageUris\":[\"http://schema.mathworks.com/mf0/Connector/R2020b\"],\"version\":\"1.0\"}"
  Divide : Product  Inputs=/*
  "Nernst’s Eq " : Subsystem
      settings: PortSchema="{\"entries\":[{\"content\":{\"sides\":[{\"content\":{\"connectorIds\":[\"In1\",\"In2\",\"In3\"]},\"type\":\"ConnectorPlacement.EquallySpacedRectSide\",\"uuid\":\"1b300774-e64d-4a8a-a2e9-ecdc71723fee\"},{\"content\":{\"connectorIds\":[\"Out1\"],\"side\":\"RIGHT\"},\"type\":\"ConnectorPlacement.EquallySpacedRectSide\",\"uuid\":\"354a04f1-cc66-4a63-8c50-8080316e29e9\"},{\"content\":{\"connectorIds\":[\"In4\"],\"side\":\"TOP\"},\"type\":\"ConnectorPlacement.EquallySpacedRectSide\",\"uuid\":\"b48b7bda-dd37-468f-ab7d-ccd563a69f0b\"}]},\"type\":\"ConnectorPlacement.EquallySpacedConnector\",\"uuid\":\"ddfd4041-6e53-4893-9028-34e5ff9f82d6\"}],\"packageUris\":[\"http://schema.mathworks.com/mf0/Connector/R2020b\"],\"version\":\"1.0\"}"
  Scope : Scope
  Subsystem : Subsystem
  Sum of Elements : Sum  Inputs=+
  Sum of Elements1 : Sum  Inputs=+
  pa : Outport
  va : Outport  Port=2
  vc : Outport  Port=3
  pc : Outport  Port=4
  Voltaje : Outport  Port=5
  wires:
  Air[mol/s]/1 -> Subsystem/1(Air[mol/s])
  Anode/1(pa) -> pa/1  "pa"
  Anode/2(pa_out) -> va/1  "pa_out"
  Cathode/1(pc) -> pc/1  "pc"
  Subsystem/1(Cathode [mol/s]) -> Sum of Elements1/1, Cathode/1(qc_in)  "qin_cath"
  Cathode/3(pc_O2) -> Anode/3(pc_O2)
  Cathode/2(pc_out) -> vc/1  "pc_out"
  I/1 -> Cathode/2(I), "Nernst’s Eq "/2(I), Anode/2(I)
  T/1 -> Cathode/3(T), "Nernst’s Eq "/3(T), Anode/4(T)
  qin_anode/1 -> Scope/1, Anode/1(qa_in), Sum of Elements/1
  "Nernst’s Eq "/1(V) -> Voltaje/1  "V"
  Anode/3(la) -> "Nernst’s Eq "/1(Xa)
  Sum of Elements/1 -> [fanode]
  Sum of Elements1/1 -> [fcathode]
  [fanode] -> Divide/1
  [fcathode] -> Divide/2
  Divide/1 -> "Nernst’s Eq "/4(ratio a/c)

== system crop_simulation/Control Systems/Heater/SOFC cascada/Water Tank /Control Law/Control Flow Rate [%] ==
  Ti : Inport
  Constant : Constant  Value=parameters.Tref
  Minus : Sum  Inputs=+-
  PID Controller : pid_lib/PID Controller  Controller=PID  Form=Parallel  TimeDomain=Continuous-time  UseExternalTs=off  SampleTime=-1  IntegratorMethod=Forward Euler  FilterMethod=Forward Euler  ControllerParametersSource=internal  P=1.5  I=1  D=0  UseFilter=on  N=100  TunerSelectOption=Transfer Function Based (PID Tuner App)  InitialConditionSource=internal  InitialConditionForIntegrator=0  InitialConditionForFilter=0  DifferentiatorICPrevScaledInput=0  ExternalReset=none  TrackingMode=off  Kt=1  LimitOutput=on  SatLimitsSource=internal  UpperSaturationLimit=1  LowerSaturationLimit=0  LinearizeAsGain=on  AntiWindupMode=clamping  Kb=1  POutMin=[]  POutMax=[]  IOutMin=[]  IOutMax=[]  DOutMin=[]  DOutMax=[]  NOutMin=[]  NOutMax=[]  SumOutMin=[]  SumOutMax=[]  SaturationOutMin=[]  SaturationOutMax=[]  PParamMin=[]  PParamMax=[]  IParamMin=[]  IParamMax=[]  DParamMin=[]  DParamMax=[]  NParamMin=[]  NParamMax=[]  KbParamMin=[]  KbParamMax=[]  KtParamMin=[]  KtParamMax=[]  KbOutMin=[]  KbOutMax=[]  KtOutMin=[]  KtOutMax=[]  IntegratorOutMin=[]  IntegratorOutMax=[]  FilterOutMin=[]  FilterOutMax=[]  SumI1OutMin=[]  SumI1OutMax=[]  SumI2OutMin=[]  SumI2OutMax=[]  SumI3OutMin=[]  SumI3OutMax=[]  SumI4OutMin=[]  SumI4OutMax=[]  SumDOutMin=[]  SumDOutMax=[]  DifferentiatorOutMin=[]  DifferentiatorOutMax=[]  FilterDiffOutCoefMin=[]  FilterDiffOutCoefMax=[]  ReciprocalOutMin=[]  ReciprocalOutMax=[]  SumDenOutMin=[]  SumDenOutMax=[]  SumNumOutMin=[]  SumNumOutMax=[]  DivideOutMin=[]  DivideOutMax=[]  UdiffTsProdOutMin=[]  UdiffTsProdOutMax=[]  NTsProdOutMin=[]  NTsProdOutMax=[]  UintegralTsProdOutMin=[]  UintegralTsProdOutMax=[]  UngainTsProdOutMin=[]  UngainTsProdOutMax=[]  IntegratorContinuousStateAttributes=''  IntegratorStateMustResolveToSignalObject=off  IntegratorRTWStateStorageClass=Auto  FilterContinuousStateAttributes=''  FilterStateMustResolveToSignalObject=off  FilterRTWStateStorageClass=Auto  ParallelPVariant=InternalParameters  IdealPVariant=Disabled  IVariant=InternalParameters  DVariant=InternalParameters  IntegratorVariant=Continuous  SatVariant=Enabled  AWVariant=ContClampingParallel  PCopyVariant=Disabled  TRVariant=Disabled  FdbkBlocksVariant=Forward  IdealPFdbkVariant=Disabled  SatFdbkVariant=Disabled  DerivativeFilterVariant=ContFilter  NVariant=InternalParameters  NCopyVariant=Disabled  FilterICVariant=InternalICsFilter  IntegratorICVariant=InternalICs  ExternalResetVariant=Disabled  TRSumVariant=Passthrough  SumFdbkVariant=Disabled  SumVariant=Sum_PID  TsampFilterVariant=InternalTs  TsampNgainVariant=Passthrough  TsampIntegralVariant=Passthrough  ExternalSaturationOutDataTypeStr=Inherit: Same as second input
  Scope : Scope  NumInputPorts=2
  Out1 : Outport
  wires:
  Constant/1 -> Scope/1, Minus/1
  Minus/1 -> PID Controller/1
  Ti/1 -> Scope/2, Minus/2
  PID Controller/1 -> Out1/1

== system crop_simulation/Control Systems/Heater/SOFC/Control OP/Select Operation Point/Select Operation Point/If Action Subsystem ==
  Action Port : ActionPort  ActionPortLabel=if(u1 < 20)
  Constant : Constant  Value=4
  Out1 : Outport
  wires:
  Constant/1 -> Out1/1

== system crop_simulation/Control Systems/Heater/SOFC/Control OP/Select Operation Point/Select Operation Point/If Action Subsystem1 ==
  Action Port : ActionPort  ActionPortLabel=elseif((u1 >= 20)&(u1<50))
  Constant : Constant  Value=3
  Out1 : Outport
  wires:
  Constant/1 -> Out1/1

== system crop_simulation/Control Systems/Heater/SOFC/Control OP/Select Operation Point/Select Operation Point/If Action Subsystem2 ==
  Action Port : ActionPort  ActionPortLabel=elseif(u1>=50)
  Constant : Constant
  Out1 : Outport
  wires:
  Constant/1 -> Out1/1

== system crop_simulation/Control Systems/Heater/SOFC/Control OP/Transformacion Flujos/If Action Subsystem/Subsystem ==
  Constant : Constant  Value=11.64
  Constant1 : Constant  Value=14.14
  Constant2 : Constant  Value=36.18
  Constant3 : Constant  Value=144
  Out Bus Element : Outport  PortName=OP  Element=Diesel [ml/min]
  Out Bus Element1 : Outport  PortName=OP  Element=Steam [ml/min]
  Out Bus Element2 : Outport  PortName=OP  Element=Air [NL/min]
  Out Bus Element3 : Outport  PortName=OP  Element=Air_cath [NL/min]
  wires:
  Constant1/1 -> Out Bus Element1/1
  Constant2/1 -> Out Bus Element2/1
  Constant/1 -> Out Bus Element/1
  Constant3/1 -> Out Bus Element3/1

== system crop_simulation/Control Systems/Heater/SOFC/Control OP/Transformacion Flujos/If Action Subsystem1/Subsystem1 ==
  Constant : Constant  Value=7.83
  Constant1 : Constant  Value=9.51
  Constant2 : Constant  Value=24.34
  Constant3 : Constant  Value=96
  Out Bus Element : Outport  PortName=OP  Element=Diesel [ml/min]
  Out Bus Element1 : Outport  PortName=OP  Element=Steam [ml/min]
  Out Bus Element2 : Outport  PortName=OP  Element=Air [NL/min]
  Out Bus Element3 : Outport  PortName=OP  Element=Air_cath [NL/min]
  wires:
  Constant1/1 -> Out Bus Element1/1
  Constant2/1 -> Out Bus Element2/1
  Constant/1 -> Out Bus Element/1
  Constant3/1 -> Out Bus Element3/1

== system crop_simulation/Control Systems/Heater/SOFC/Control OP/Transformacion Flujos/If Action Subsystem2/Subsystem2 ==
  Constant : Constant  Value=6.51
  Constant1 : Constant  Value=7.91
  Constant2 : Constant  Value=20.24
  Constant3 : Constant  Value=80
  Out Bus Element : Outport  PortName=OP  Element=Diesel [ml/min]
  Out Bus Element1 : Outport  PortName=OP  Element=Steam [ml/min]
  Out Bus Element2 : Outport  PortName=OP  Element=Air [NL/min]
  Out Bus Element3 : Outport  PortName=OP  Element=Air_cath [NL/min]
  wires:
  Constant1/1 -> Out Bus Element1/1
  Constant2/1 -> Out Bus Element2/1
  Constant/1 -> Out Bus Element/1
  Constant3/1 -> Out Bus Element3/1

== system crop_simulation/Control Systems/Heater/SOFC/Control OP/Transformacion Flujos/If Action Subsystem3/Subsystem2 ==
  Constant : Constant  Value=4.41
  Constant1 : Constant  Value=5.36
  Constant2 : Constant  Value=13.72
  Constant3 : Constant  Value=55
  Out Bus Element : Outport  PortName=OP  Element=Diesel [ml/min]
  Out Bus Element1 : Outport  PortName=OP  Element=Steam [ml/min]
  Out Bus Element2 : Outport  PortName=OP  Element=Air [NL/min]
  Out Bus Element3 : Outport  PortName=OP  Element=Air_cath [NL/min]
  wires:
  Constant1/1 -> Out Bus Element1/1
  Constant2/1 -> Out Bus Element2/1
  Constant/1 -> Out Bus Element/1
  Constant3/1 -> Out Bus Element3/1

== system crop_simulation/Control Systems/Heater/SOFC/Reformer  - SOFC System/Reformer /Subsystem/Order Data ==
  note: Target
  note: Target
  note: 'H2' , 'O2' , 'H2O' , 'N2' , 'CO' , 'CH4' , 'CO2' , 'Diesel' ,'Ar','Csoot'
  In1 : Inport
  Demux : Demux  Outputs=8
  Vector Concatenate : Concatenate  NumInputs=10
  Out1 : Outport
  wires:
  In1/1 -> Demux/1
  Demux/1 -> [Ar]
  Demux/2 -> [CH4]
  Demux/3 -> [CO]
  Demux/4 -> [CO2]
  Demux/5 -> [H2]
  Demux/6 -> [H2O]
  Demux/7 -> [N2]
  Demux/8 -> [Csoot]
  [H2] -> Vector Concatenate/1
  [H2O] -> Vector Concatenate/3
  [N2] -> Vector Concatenate/4
  [CO] -> Vector Concatenate/5
  [CH4] -> Vector Concatenate/6
  [CO2] -> Vector Concatenate/7
  [Ar] -> Vector Concatenate/9
  [Csoot] -> Vector Concatenate/10
  Vector Concatenate/1 -> Out1/1

== system crop_simulation/Control Systems/Heater/SOFC/Reformer  - SOFC System/Reformer /Subsystem/Order Data1 ==
  note: 'H2' , 'O2' , 'H2O' , 'N2' , 'CO' , 'CH4' , 'CO2' , 'Diesel' ,'Ar','Csoot'
  In1 : Inport
  Demux : Demux  Outputs=6
  Vector Concatenate : Concatenate  NumInputs=10
  Out1 : Outport
  wires:
  In1/1 -> Demux/1
  Demux/1 -> [N2]
  Demux/2 -> [O2]
  Demux/3 -> [CO2]
  Demux/4 -> [H2O]
  Demux/5 -> [Ar]
  Demux/6 -> [Diesel]
  [H2O] -> Vector Concatenate/3
  [N2] -> Vector Concatenate/4
  [CO2] -> Vector Concatenate/7
  [Ar] -> Vector Concatenate/9
  Vector Concatenate/1 -> Out1/1
  [O2] -> Vector Concatenate/2
  [Diesel] -> Vector Concatenate/8

== system crop_simulation/Control Systems/Heater/SOFC/Reformer  - SOFC System/Reformer /Subsystem/Subsystem ==
  In1 : Inport
  Subsystem : Subsystem  VariantControl=Choice
  Subsystem1 : Subsystem  VariantControl=Choice_1
  Out1 : Outport

== system crop_simulation/Control Systems/Heater/SOFC/Reformer  - SOFC System/Reformer /Subsystem/Subsystem1 ==
  In1 : Inport
  Subsystem : Subsystem  VariantControl=Choice_1
  Subsystem1 : Subsystem  VariantControl=Choice
  Out1 : Outport

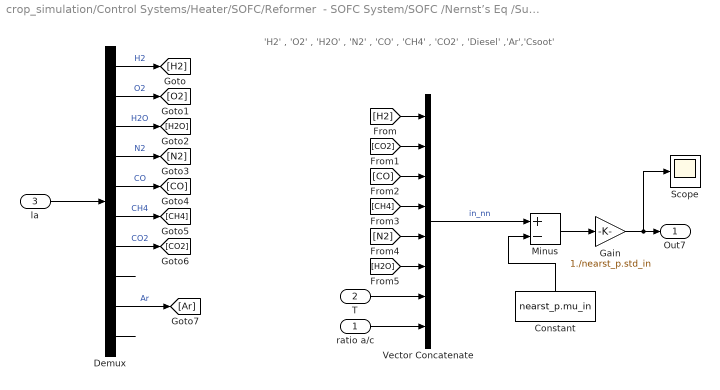
== system crop_simulation/Control Systems/Heater/SOFC/Reformer  - SOFC System/SOFC /Nernst’s Eq /Subsystem ==
  note: 'H2' , 'O2' , 'H2O' , 'N2' , 'CO' , 'CH4' , 'CO2' , 'Diesel' ,'Ar','Csoot'
  ratio a/c : Inport
  T : Inport  Port=2
  la : Inport  Port=3
  Constant : Constant  Value=nearst_p.mu_in
  Demux : Demux  Outputs=10
  Gain : Gain  Gain=1./nearst_p.std_in
  Minus : Sum  Inputs=+-
  Scope : Scope
  Vector Concatenate : Concatenate  NumInputs=8
  Out7 : Outport
  wires:
  Demux/7 -> [CO2]  "CO2"
  la/1 -> Demux/1
  Demux/3 -> [H2O]  "H2O"
  Demux/1 -> [H2]  "H2"
  Demux/8 -> ?
  Demux/2 -> [O2]  "O2"
  Demux/10 -> ?
  Demux/9 -> [Ar]  "Ar"
  Demux/5 -> [CO]  "CO"
  Demux/4 -> [N2]  "N2"
  Demux/6 -> [CH4]  "CH4"
  ratio a/c/1 -> Vector Concatenate/8
  T/1 -> Vector Concatenate/7
  [H2] -> Vector Concatenate/1
  [CO2] -> Vector Concatenate/2
  [CO] -> Vector Concatenate/3
  [CH4] -> Vector Concatenate/4
  [N2] -> Vector Concatenate/5
  [H2O] -> Vector Concatenate/6
  Vector Concatenate/1 -> Minus/1  "in_nn"
  Constant/1 -> Minus/2
  Minus/1 -> Gain/1
  Gain/1 -> Scope/1, Out7/1

== system crop_simulation/Control Systems/Heater/SOFC/Reformer  - SOFC System/SOFC /Nernst’s Eq /Subsystem1 ==
  In1 : Inport
  Subsystem : Subsystem  VariantControl=Choice_1
  Subsystem1 : Subsystem  VariantControl=Choice
  Out1 : Outport

== system crop_simulation/Control Systems/Heater/SOFC cascada/Control Operations Points/Control OP/Select Operation Point/Relay ==
  Error [ºC] : Inport
  Relay : Relay  OnSwitchValue=80  OffSwitchValue=20  OnOutputValue=2  OffOutputValue=4
  OP : Outport
  wires:
  Error [ºC]/1 -> Relay/1
  Relay/1 -> OP/1

== system crop_simulation/Control Systems/Heater/SOFC cascada/Control Operations Points/Control OP/Select Operation Point/Relay 3 ==
  Error [ºC] : Inport
  Delay : Delay  DelayLength=1  InitialCondition=1
  Delay1 : Delay  DelayLength=1  InitialCondition=1
  MATLAB Function : MATLAB Function  TreatAsAtomicUnit=on
  Rate Transition : RateTransition  InitialCondition=10  OutPortSampleTime=1/(60*24)
  OP : Outport
  wires:
  MATLAB Function/1(next_state) -> Delay/1, OP/1
  Delay/1 -> MATLAB Function/3(state)
  Error [ºC]/1 -> Rate Transition/1
  Rate Transition/1 -> Delay1/1, MATLAB Function/2(Error)
  Delay1/1 -> MATLAB Function/1(Pre_Error)

== system crop_simulation/Control Systems/Heater/SOFC cascada/Control Operations Points/Control OP/Select Operation Point/Select Operation Point ==
  Error [ºC] : Inport
  If : If  IfExpression=u1 < 20  ElseIfExpressions=(u1 >= 20)&(u1<50),u1>=50  ShowElse=off  ZeroCross=off
  If Action Subsystem : Subsystem  TreatAsAtomicUnit=on
  If Action Subsystem1 : Subsystem  TreatAsAtomicUnit=on
  If Action Subsystem2 : Subsystem  TreatAsAtomicUnit=on
  Merge : Merge  Inputs=3
  OP : Outport
  wires:
  Error [ºC]/1 -> If/1
  If Action Subsystem1/1(Out1) -> Merge/2
  Merge/1 -> OP/1
  If/3 -> If Action Subsystem2/Action
  If/1 -> If Action Subsystem/Action
  If Action Subsystem2/1(Out1) -> Merge/3
  If Action Subsystem/1(Out1) -> Merge/1
  If/2 -> If Action Subsystem1/Action

== system crop_simulation/Control Systems/Heater/SOFC cascada/Control Operations Points/Control OP/Transformacion Flujos/If Action Subsystem ==
  Action Port : ActionPort  ActionPortLabel=case [ 4 ]:
  Subsystem : Subsystem
  Out1 : Outport
  wires:
  Subsystem/1(OP) -> Out1/1

== system crop_simulation/Control Systems/Heater/SOFC cascada/Control Operations Points/Control OP/Transformacion Flujos/If Action Subsystem1 ==
  Action Port : ActionPort  ActionPortLabel=case [ 3 ]:
  Subsystem1 : Subsystem
  Out1 : Outport
  wires:
  Subsystem1/1(OP) -> Out1/1

== system crop_simulation/Control Systems/Heater/SOFC cascada/Control Operations Points/Control OP/Transformacion Flujos/If Action Subsystem2 ==
  Action Port : ActionPort  ActionPortLabel=case [ 2 ]:
  Subsystem2 : Subsystem
  Out1 : Outport
  wires:
  Subsystem2/1(OP) -> Out1/1

== system crop_simulation/Control Systems/Heater/SOFC cascada/Control Operations Points/Control OP/Transformacion Flujos/If Action Subsystem3 ==
  Action Port : ActionPort  ActionPortLabel=case [ 1 ]:
  Subsystem2 : Subsystem
  Out1 : Outport
  wires:
  Subsystem2/1(OP) -> Out1/1

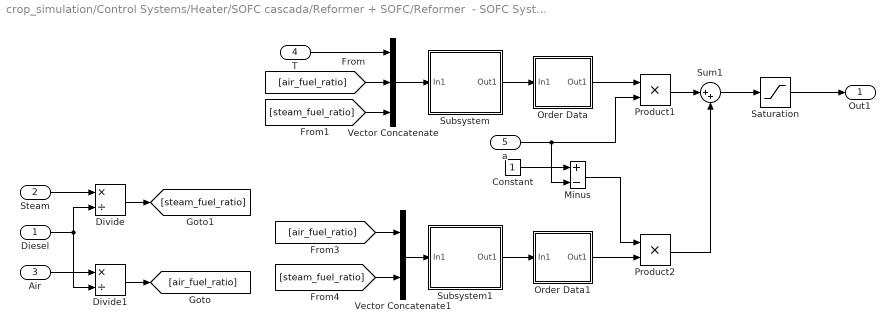
== system crop_simulation/Control Systems/Heater/SOFC cascada/Reformer + SOFC/Reformer  - SOFC System/Reformer /Subsystem ==
  Diesel : Inport
  Steam : Inport  Port=2
  Air : Inport  Port=3
  T : Inport  Port=4
  a : Inport  Port=5
  Constant : Constant
  Divide : Product  Inputs=*/
  Divide1 : Product  Inputs=*/
  Minus : Sum  Inputs=+-
  Order Data : Subsystem
  Order Data1 : Subsystem
  Product1 : Product
  Product2 : Product
  Saturation : Saturate  UpperLimit=inf  LowerLimit=0
  Subsystem : Subsystem  Variant=on  VariantControlMode=label  VariantControl=Choice  LabelModeActiveChoice=Choice_1
  Subsystem1 : Subsystem  Variant=on  VariantControlMode=label  VariantControl=Choice  LabelModeActiveChoice=Choice_1
  Sum1 : Sum  Inputs=|++
  Vector Concatenate : Concatenate  NumInputs=3
  Vector Concatenate1 : Concatenate
  Out1 : Outport
  wires:
  a/1 -> Product1/2, Minus/2
  [steam_fuel_ratio] -> Vector Concatenate/3
  Product1/1 -> Sum1/1
  T/1 -> Vector Concatenate/1
  [air_fuel_ratio] -> Vector Concatenate1/1
  Product2/1 -> Sum1/2
  [steam_fuel_ratio] -> Vector Concatenate1/2
  Order Data1/1(Out1) -> Product2/2
  Minus/1 -> Product2/1
  Order Data/1(Out1) -> Product1/1
  [air_fuel_ratio] -> Vector Concatenate/2
  Constant/1 -> Minus/1
  Steam/1 -> Divide/1
  Diesel/1 -> Divide1/2, Divide/2
  Air/1 -> Divide1/1
  Divide/1 -> [steam_fuel_ratio]
  Divide1/1 -> [air_fuel_ratio]
  Saturation/1 -> Out1/1
  Sum1/1 -> Saturation/1
  Vector Concatenate/1 -> Subsystem/1(In1)
  Subsystem/1(Out1) -> Order Data/1(In1)
  Vector Concatenate1/1 -> Subsystem1/1(In1)
  Subsystem1/1(Out1) -> Order Data1/1(In1)

== system crop_simulation/Control Systems/Heater/SOFC cascada/Reformer + SOFC/Reformer  - SOFC System/Reformer /Subsystem1 ==
  Mass Flow : Inport
  T : Inport  Port=2
  Ainhoa : Subsystem  VariantControl=Choice_1
  Simple : Subsystem  VariantControl=Choice
  activity : Outport

== system crop_simulation/Control Systems/Heater/SOFC cascada/Reformer + SOFC/Reformer  - SOFC System/SOFC /Anode ==
  qa_in : Inport
  I : Inport  Port=2
  pc_O2 : Inport  Port=3
  T : Inport  Port=4
  Divide2 : Product  Inputs=**
  Gain : Gain  Gain=p.ValveConstants_an
  Gain1 : Gain  Gain=p.N0
  Gain2 : Gain  Gain=p.R/p.Vanode
  Integrator : Integrator  InitialCondition=x0.pa  LowerSaturationLimit=0  ZeroCross=off
  MATLAB Function : MATLAB Function  TreatAsAtomicUnit=on
  Scope : Scope
  Scope1 : Scope
  Scope2 : Scope
  Sum : Sum  Inputs=+-+
  seconds 2 days : Gain  Gain=3600*24
  pa : Outport
  pa_out : Outport  Port=2
  la : Outport  Port=3
  wires:
  Sum/1 -> Divide2/1
  Integrator/1 -> Scope/1, Gain/1, MATLAB Function/4(pa), pa/1
  Gain2/1 -> Divide2/2
  qa_in/1 -> Sum/1, MATLAB Function/1(qa_in)
  Gain/1 -> pa_out/1, Sum/2
  I/1 -> MATLAB Function/2(I)
  T/1 -> Gain2/1
  MATLAB Function/2(la) -> la/1, Scope1/1
  pc_O2/1 -> MATLAB Function/3(pc_O2)
  MATLAB Function/1(ra) -> Gain1/1
  Gain1/1 -> Scope2/1, Sum/3
  Divide2/1 -> seconds 2 days/1
  seconds 2 days/1 -> Integrator/1

== system crop_simulation/Control Systems/Heater/SOFC cascada/Reformer + SOFC/Reformer  - SOFC System/SOFC /Cathode ==
  qc_in : Inport
  I : Inport  Port=2
  T : Inport  Port=3
  Divide3 : Product  Inputs=**
  Gain1 : Gain  Gain=p.N0
  Gain2 : Gain  Gain=p.R/p.Vcatho
  Integrator1 : Integrator  InitialCondition=x0.pc  LowerSaturationLimit=0  ZeroCross=off
  MATLAB Function : MATLAB Function  TreatAsAtomicUnit=on
  Scope : Scope
  Scope1 : Scope  NumInputPorts=2
  Selector : Selector  InputPortWidth=10  IndexOptions=Index vector (dialog)  Indices=2  OutputSizes=1
  Sum1 : Sum  Inputs=+-+
  seconds 2 days : Gain  Gain=3600*24
  valve : Gain  Gain=p.ValveConstants_cath
  pc : Outport
  pc_out : Outport  Port=2  Unit=mol/s
  pc_O2 : Outport  Port=3
  wires:
  Sum1/1 -> Divide3/1
  Integrator1/1 -> Selector/1, valve/1, Scope/1, pc/1
  qc_in/1 -> Sum1/1
  Gain2/1 -> Divide3/2
  T/1 -> Gain2/1
  valve/1 -> Sum1/2, pc_out/1
  I/1 -> Scope1/1, MATLAB Function/1(I)
  MATLAB Function/1(rc) -> Gain1/1
  Gain1/1 -> Sum1/3
  Divide3/1 -> seconds 2 days/1
  seconds 2 days/1 -> Integrator1/1
  Selector/1 -> pc_O2/1, Scope1/2, MATLAB Function/2(pc_O2)
